simulink model "testemplanner_cs_old"  (R2020b)
settings: Solver=FixedStepAuto  StartTime=0.0  StopTime=50  FixedStep=1/1000  MaxStep=3  RelTol=1e-3
PreLoadFcn:
  | mbxruntime.callbacks.PreLoadFcn(bdroot);
PostLoadFcn:
  | mbxruntime.callbacks.PostLoadFcn(bdroot);
InitFcn:
  | mbxruntime.callbacks.InitFcn(bdroot);
StartFcn:
  | mbxruntime.callbacks.StartFcn(bdroot);
StopFcn:
  | mbxruntime.callbacks.StopFcn(bdroot);
model workspace (MAT data in the model file):
  mbox_table : object (value not decoded)
  model_closed = 0
  sim_status = 0
values from neighbouring files (symbols this model uses):
  c_factor = 43.75    [emplanner_init.m]
  cf = -175016    [emplanner_init.m]
  cr = -130634    [emplanner_init.m]
  global_path_x = [-8.9703 -7.97092389706 -6.97280725051 -5.97596683104 -4.98040839797 -3.98613358222 -2.99314248891 -2.0014346597 -1.01100942869 -0.0218660539602 0.965996233729 1.95257821297 ... (3001 elements, 3001x1)]    [global_path.mat]
  global_path_y = [9.935 9.935 9.935 9.935 9.935 9.935 9.935 9.935 9.935 9.935 9.935 9.935 ... (3001 elements, 3001x1)]    [global_path.mat]
  KD_PID_distance = 0.0    (= 0)    [emplanner_init.m]
  KD_PID_speed = 0    [emplanner_init.m]
  KI_PID_distance = 0.0    (= 0)    [emplanner_init.m]
  KI_PID_speed = 0    [emplanner_init.m]
  KP_PID_distance = 0.5    [emplanner_init.m]
  KP_PID_speed = 1.8    [emplanner_init.m]
  la = 1.265    [emplanner_init.m]
  lb = 2.947-1.265    (= 1.682)    [emplanner_init.m]
  LQR_K1 = k(:,1)'    [emplanner_init.m]
  LQR_K2 = k(:,2)'    [emplanner_init.m]
  LQR_K3 = k(:,3)'    [emplanner_init.m]
  LQR_K4 = k(:,4)'    [emplanner_init.m]
  m = 2020    [emplanner_init.m]
  rack_displacement = [-39.14 , -37.2 , -35.29 , -33.43 , -31.6 , -29.81 , -28.06 , -26.34 , -24.66 ,      -23.01 , -21.38 , -19.79 , -18.23 , -16.69 , -15.18 , -13.7 , -12.23 , -10.8 , -9.38 , -7.98 ,     -6.61 , -5.25 , -3.91 , -2.59 , -1.29 , 0 , 1.27 , 2.54 , 3.78 , 5.02 , 6.24 , 7.46 , 8.66 ,      9.86 , 11.05 , 12.24 , 13.41 , 14.59 , 15.76 , 16.92 , 18.09 , 19.25 , 20.42 , 21.59 , 22.76 ,      23.93 , 25.11 , 26 ...(+26 chars)    [emplanner_init.m]
  right_wheel_ground = [-70 ,-67.2 , -64.4 , -61.6 , -58.8 , -56 , -53.2 , -50.4 , -47.6 , -44.8 , -42 ,      -39.2 , -36.4 , -33.6 , -30.8 , -28 , -25.2 , -22.4 , -19.6 , -16.8 , -14 , -11.2 , -8.4 , -5.6 ,      -2.8 , 0 , 2.8 , 5.6 , 8.4 , 11.2 , 14 , 16.8 , 19.6 , 22.4 , 25.2 , 28 , 30.8 , 33.6 , 36.4 ,      39.2 , 42 , 44.8 , 47.6 , 50.4 , 53.2 , 56 , 58.8 , 61.6 , 64.4 , 67.2 , 70 ]    [emplanner_init.m]
  vx_break_point = zeros(1,5000)    [emplanner_init.m]
undefined symbols (not defined in the file or in its folder): aubr, DiscIntNeverNeededParam, tablebr, vubr, warningInitialVelocity, x0
libraries: PreScanSimulinkLibrary x33, simulink x19, simulink_extras x10, Solver_SF x1
(part 6 of 12)

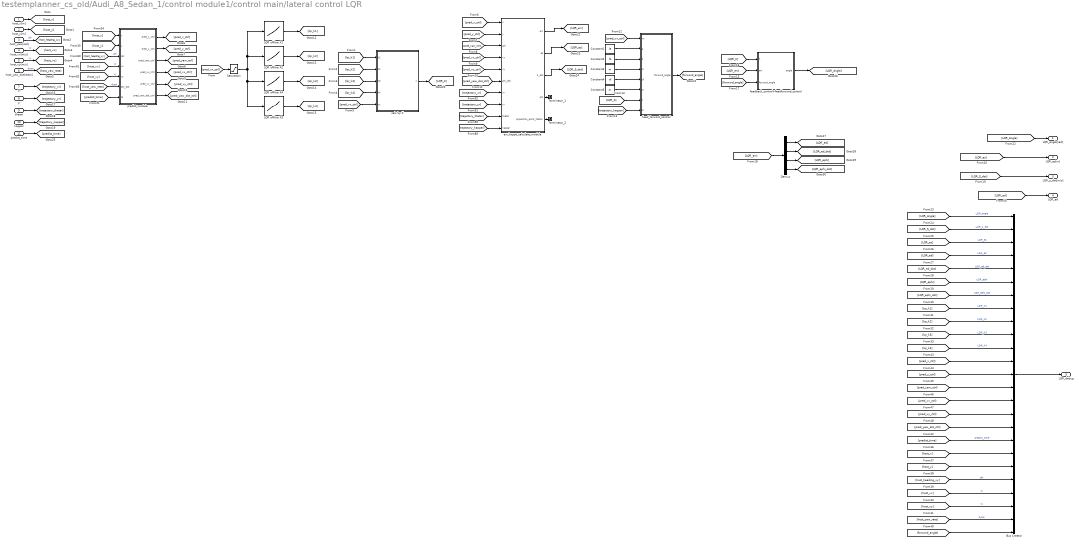
== system testemplanner_cs_old/Audi_A8_Sedan_1/control module1/control main/lateral control LQR ==
  host_x[m] : Inport
  host_y[m] : Inport  Port=2
  host_yaw[rad] : Inport  Port=3
  host_vx[m/s] : Inport  Port=4
  host_vy[m/s] : Inport  Port=5
  host_yaw_dot[rad/s] : Inport  Port=6
  xr : Inport  Port=7
  yr : Inport  Port=8
  thetar : Inport  Port=9
  kappar : Inport  Port=10
  predict_time : Inport  Port=11
  Bus Creator : BusCreator  Inputs=25
  Constant1 : Constant  Value=la
  Constant2 : Constant  Value=lb
  Constant3 : Constant  Value=m
  Constant4 : Constant  Value=cf
  Constant5 : Constant  Value=cr
  Demux : Demux
  LQR offline K1 : Lookup_n-D  NumberOfTableDimensions=1  BreakpointsForDimension1=vx_break_point  Table=LQR_K1  InternalRulePriority=Speed  RndMeth=Simplest  InputSameDT=on
  LQR offline K2 : Lookup_n-D  NumberOfTableDimensions=1  BreakpointsForDimension1=vx_break_point  Table=LQR_K2  InternalRulePriority=Speed  RndMeth=Simplest  InputSameDT=on
  LQR offline K3 : Lookup_n-D  NumberOfTableDimensions=1  BreakpointsForDimension1=vx_break_point  Table=LQR_K3  InternalRulePriority=Speed  RndMeth=Simplest  InputSameDT=on
  LQR offline K4 : Lookup_n-D  NumberOfTableDimensions=1  BreakpointsForDimension1=vx_break_point  Table=LQR_K4  InternalRulePriority=Speed  RndMeth=Simplest  InputSameDT=on
  Saturation : Saturate  UpperLimit=50  LowerLimit=0
  Terminator_1 : Terminator
  Terminator_2 : Terminator
  calc lqr K : MATLAB Function  TreatAsAtomicUnit=on
  err_kappa_calculate_module : MATLAB Function  TreatAsAtomicUnit=on
  feed_forword_control : MATLAB Function  TreatAsAtomicUnit=on
  feedback_control+feedforword_control : MATLAB Function  TreatAsAtomicUnit=on
  predict_module : MATLAB Function  TreatAsAtomicUnit=on
  LQR_angle[rad] : Outport  VectorParamsAs1DForOutWhenUnconnected=off
  LQR_es[m] : Outport  Port=2  VectorParamsAs1DForOutWhenUnconnected=off
  LQR_s_dot[m/s] : Outport  Port=3  VectorParamsAs1DForOutWhenUnconnected=off
  LQR_ed : Outport  Port=4  VectorParamsAs1DForOutWhenUnconnected=off
  LQR_debug : Outport  Port=5  VectorParamsAs1DForOutWhenUnconnected=off
  wires:
  [host_vy] -> predict_module/5(vy)  "vy"
  [host_x] -> predict_module/1(x)
  [host_yaw_rate] -> predict_module/6(phi_dot)  "dyaw"
  [host_vx] -> predict_module/4(vx)  "vx"
  [host_y] -> predict_module/2(y)
  [host_heading_xy] -> predict_module/3(phi)  "phi"
  [predict_time] -> predict_module/7(ts)
  host_x[m]/1 -> [host_x]
  host_y[m]/1 -> [host_y]
  host_yaw[rad]/1 -> [host_heading_xy]  "phi"
  host_vx[m/s]/1 -> [host_vx]  "vx"
  host_vy[m/s]/1 -> [host_vy]  "vy"
  host_yaw_dot[rad/s]/1 -> [host_yaw_rate]  "dyaw"
  predict_module/1(pred_x_ctrl) -> [pred_x_ctrl]
  predict_module/2(pred_y_ctrl) -> [pred_y_ctrl]
  predict_module/3(pred_yaw_ctrl) -> [pred_yaw_ctrl]
  predict_module/4(pred_vx_ctrl) -> [pred_vx_ctrl]
  predict_module/5(pred_vy_ctrl) -> [pred_vy_ctrl]
  predict_module/6(pred_yaw_dot_ctrl) -> [pred_yaw_dot_ctrl]
  [pred_vx_ctrl] -> Saturation/1
  LQR offline K1/1 -> [lqr_k1]
  LQR offline K2/1 -> [lqr_k2]
  LQR offline K4/1 -> [lqr_k3]
  LQR offline K3/1 -> [lqr_k4]
  [pred_vx_ctrl] -> calc lqr K/5(vx)
  [lqr_k4] -> calc lqr K/4(k4)
  [lqr_k3] -> calc lqr K/3(k3)
  [lqr_k2] -> calc lqr K/2(k2)
  [lqr_k1] -> calc lqr K/1(k1)
  [pred_x_ctrl] -> err_kappa_calculate_module/1(x)
  [pred_y_ctrl] -> err_kappa_calculate_module/2(y)
  [pred_yaw_ctrl] -> err_kappa_calculate_module/3("phi ")
  [pred_vx_ctrl] -> err_kappa_calculate_module/4(vx)
  [pred_vy_ctrl] -> err_kappa_calculate_module/5(vy)
  [pred_yaw_dot_ctrl] -> err_kappa_calculate_module/6(phi_dot)
  xr/1 -> [trajectory_xr]
  yr/1 -> [trajectory_yr]
  thetar/1 -> [trajectory_thetar]
  kappar/1 -> [trajectory_kappar]
  [trajectory_xr] -> err_kappa_calculate_module/7(xr)
  [trajectory_yr] -> err_kappa_calculate_module/8(yr)
  [trajectory_kappar] -> err_kappa_calculate_module/10(kappar)
  [trajectory_thetar] -> err_kappa_calculate_module/9(thetar)
  [pred_vx_ctrl] -> feed_forword_control/1(vx)
  Constant1/1 -> feed_forword_control/2(a)
  Constant2/1 -> feed_forword_control/3(b)
  Constant3/1 -> feed_forword_control/4(m)
  Constant4/1 -> feed_forword_control/5(cf)
  Constant5/1 -> feed_forword_control/6(cr)
  calc lqr K/1(k) -> [LQR_K]
  [LQR_K] -> feed_forword_control/7(k)
  [trajectory_kappar] -> feed_forword_control/8(kr)
  feed_forword_control/1(forword_angle) -> [forword_angle]
  err_kappa_calculate_module/1(err) -> [LQR_err]
  [LQR_err] -> feedback_control+feedforword_control/2(err)
  [LQR_K] -> feedback_control+feedforword_control/1(k)
  [forword_angle] -> feedback_control+feedforword_control/3(forword_angle)
  [LQR_err] -> Demux/1
  err_kappa_calculate_module/2(es) -> [LQR_es]
  err_kappa_calculate_module/3(s_dot) -> [LQR_S_dot]
  [LQR_S_dot] -> LQR_s_dot[m/s]/1
  [LQR_es] -> LQR_es[m]/1
  Saturation/1 -> LQR offline K3/1, LQR offline K4/1, LQR offline K2/1, LQR offline K1/1
  predict_time/1 -> [predict_time]
  Bus Creator/1 -> LQR_debug/1
  feedback_control+feedforword_control/1(angle) -> [LQR_Angle]
  [LQR_Angle] -> LQR_angle[rad]/1
  [LQR_Angle] -> Bus Creator/1  "LQR_angle"
  [LQR_S_dot] -> Bus Creator/2  "LQR_s_dot"
  [LQR_es] -> Bus Creator/3  "LQR_es"
  Demux/1 -> [LQR_ed]
  Demux/2 -> [LQR_ed_dot]
  Demux/3 -> [LQR_ephi]
  Demux/4 -> [LQR_ephi_dot]
  [LQR_ed] -> Bus Creator/4  "LQR_ed"
  [LQR_ed_dot] -> Bus Creator/5  "LQR_ed_dot"
  [LQR_ephi] -> Bus Creator/6  "LQR_ephi"
  [LQR_ephi_dot] -> Bus Creator/7  "LQR_ephi_dot"
  [lqr_k1] -> Bus Creator/8  "LQR_K1"
  [lqr_k2] -> Bus Creator/9  "LQR_K2"
  [lqr_k3] -> Bus Creator/10  "LQR_K3"
  [lqr_k4] -> Bus Creator/11  "LQR_K4"
  [pred_x_ctrl] -> Bus Creator/12
  [pred_y_ctrl] -> Bus Creator/13
  [pred_yaw_ctrl] -> Bus Creator/14
  [pred_vx_ctrl] -> Bus Creator/15
  [pred_vy_ctrl] -> Bus Creator/16
  [pred_yaw_dot_ctrl] -> Bus Creator/17
  [predict_time] -> Bus Creator/18  "predict_time"
  [host_x] -> Bus Creator/19
  [host_y] -> Bus Creator/20
  [host_heading_xy] -> Bus Creator/21  "phi"
  [host_vx] -> Bus Creator/22  "vx"
  [host_vy] -> Bus Creator/23  "vy"
  [host_yaw_rate] -> Bus Creator/24  "dyaw"
  [forword_angle] -> Bus Creator/25
  [LQR_ed] -> LQR_ed/1
  err_kappa_calculate_module/4(phi) -> Terminator_1/1
  err_kappa_calculate_module/5(projection_point_thetar) -> Terminator_2/1

== system testemplanner_cs_old/Audi_A8_Sedan_1/control module1/control main/longitudinal control double PID ==
  s_err[m] : Inport
  speed_desire[m/s] : Inport  Port=2
  accelerate desire[m/s^2] : Inport  Port=3
  host_speed[m/s] : Inport  Port=4
  host_s_dot[m/s] : Inport  Port=5
  KP_PID_distance : Inport  Port=6
  KI_PID_distance : Inport  Port=7
  KD_PID_distance : Inport  Port=8
  KP_PID_speed : Inport  Port=9
  KI_PID_speed : Inport  Port=10
  KD_PID_speed : Inport  Port=11
  2-D Lookup Table : Lookup_n-D  BreakpointsForDimension1=vubr  BreakpointsForDimension2=aubr  Table=tablebr  InternalRulePriority=Speed  RndMeth=Simplest  InputSameDT=on
      settings: InputPortMap=u0,u1
  Add : Sum  Inputs=++-
  Add1 : Sum
  Bus Creator : BusCreator  Inputs=9
  Discrete Filter : DiscreteFilter
  MATLAB Function1 : MATLAB Function  TreatAsAtomicUnit=on
  Saturation : Saturate  UpperLimit=45  LowerLimit=-45
  Saturation1 : Saturate  UpperLimit=5  LowerLimit=-8
  discrete pid : Subsystem
  discrete pid1 : Subsystem
  throttle : Outport
  brake : Outport  Port=2
  longitudinal_debug : Outport  Port=3
  wires:
  2-D Lookup Table/1 -> MATLAB Function1/1(u)
  s_err[m]/1 -> [s_err]
  speed_desire[m/s]/1 -> [speed_desire]
  accelerate desire[m/s^2]/1 -> [accelerate_desire]
  KP_PID_distance/1 -> [KP_PID_distance]
  KI_PID_distance/1 -> [KI_PID_distance]
  KD_PID_distance/1 -> [KD_PID_distance]
  KP_PID_speed/1 -> [KP_PID_speed]
  KI_PID_speed/1 -> [KI_PID_speed]
  KD_PID_speed/1 -> [KD_PID_speed]
  [s_err] -> Discrete Filter/1
  host_speed[m/s]/1 -> [host_speed]
  [speed_desire] -> Add/2
  Add/1 -> Saturation/1
  Saturation/1 -> discrete pid1/1(err)
  discrete pid1/1(pid_out) -> Add1/1
  [accelerate_desire] -> Add1/2
  Add1/1 -> Saturation1/1
  Saturation1/1 -> 2-D Lookup Table/2
  host_s_dot[m/s]/1 -> [host_s_dot]
  [host_s_dot] -> Add/3
  [host_speed] -> 2-D Lookup Table/1
  MATLAB Function1/1(throttle) -> throttle/1
  MATLAB Function1/2(brake) -> brake/1
  [KP_PID_distance] -> Bus Creator/1  "KP_PID_distance"
  [KI_PID_distance] -> Bus Creator/2  "KI_PID_distance"
  [KD_PID_distance] -> Bus Creator/3  "KD_PID_distance"
  [KP_PID_speed] -> Bus Creator/4  "KP_PID_speed"
  [KI_PID_speed] -> Bus Creator/5  "KI_PID_speed"
  [KD_PID_speed] -> Bus Creator/6  "KD_PID_speed"
  [host_speed] -> Bus Creator/7  "host_speed"
  [s_err] -> Bus Creator/8  "s_err"
  [host_s_dot] -> Bus Creator/9  "host_s_dot"
  Bus Creator/1 -> longitudinal_debug/1
  Discrete Filter/1 -> discrete pid/1(err)
  [KP_PID_distance] -> discrete pid/2(kp)
  [KI_PID_distance] -> discrete pid/3(ki)
  [KD_PID_distance] -> discrete pid/4(kd)
  [KP_PID_speed] -> discrete pid1/2(kp)
  [KI_PID_speed] -> discrete pid1/3(ki)
  [KD_PID_speed] -> discrete pid1/4(kd)
  discrete pid/1(pid_out) -> Add/1

== system testemplanner_cs_old/Audi_A8_Sedan_1/control module1/control main/understeer compensate ==
  LQR_angle : Inport
  lateral err : Inport  Port=2
  Add : Sum  Inputs=+-
  Gain : Gain  Gain=0.01
  Manual Switch : ManualSwitch
  LQR_final_angle : Outport
  wires:
  lateral err/1 -> Gain/1
  Add/1 -> Manual Switch/2
  Manual Switch/1 -> LQR_final_angle/1
  LQR_angle/1 -> Add/1, Manual Switch/1
  Gain/1 -> Add/2

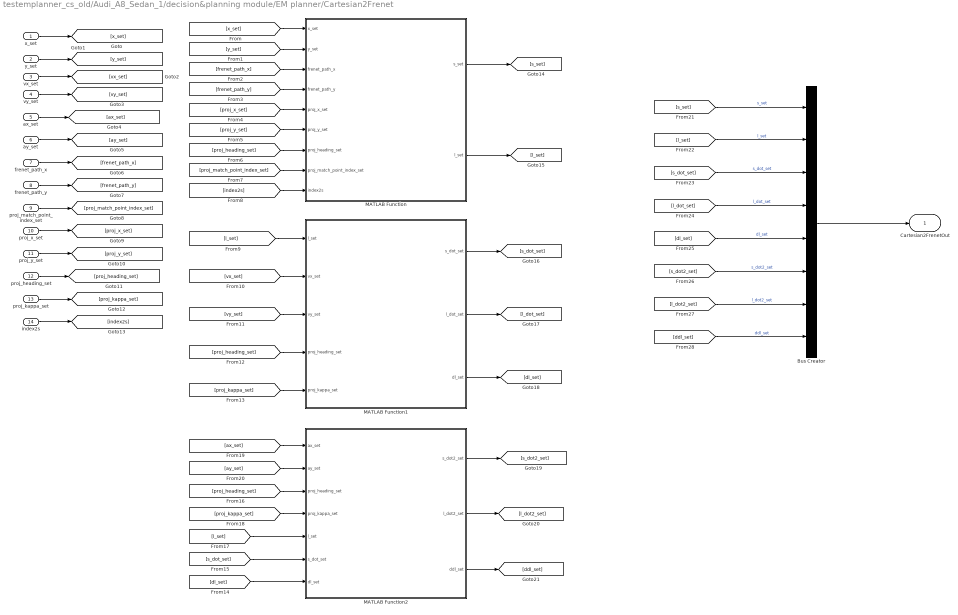
== system testemplanner_cs_old/Audi_A8_Sedan_1/decision&planning module/EM planner/Cartesian2Frenet ==
  x_set : Inport
  y_set : Inport  Port=2
  vx_set : Inport  Port=3
  vy_set : Inport  Port=4
  ax_set : Inport  Port=5
  ay_set : Inport  Port=6
  frenet_path_x : Inport  Port=7
  frenet_path_y : Inport  Port=8
  proj_match_point_index_set : Inport  Port=9
  proj_x_set : Inport  Port=10
  proj_y_set : Inport  Port=11
  proj_heading_set : Inport  Port=12
  proj_kappa_set : Inport  Port=13
  index2s : Inport  Port=14
  Bus Creator : BusCreator  Inputs=8
  MATLAB Function : MATLAB Function  TreatAsAtomicUnit=on
  MATLAB Function1 : MATLAB Function  TreatAsAtomicUnit=on
  MATLAB Function2 : MATLAB Function  TreatAsAtomicUnit=on
  Cartesian2FrenetOut : Outport
  wires:
  x_set/1 -> [x_set]
  y_set/1 -> [y_set]
  vx_set/1 -> [vx_set]
  vy_set/1 -> [vy_set]
  ax_set/1 -> [ax_set]
  ay_set/1 -> [ay_set]
  frenet_path_x/1 -> [frenet_path_x]
  frenet_path_y/1 -> [frenet_path_y]
  proj_match_point_index_set/1 -> [proj_match_point_index_set]
  proj_x_set/1 -> [proj_x_set]
  proj_y_set/1 -> [proj_y_set]
  proj_heading_set/1 -> [proj_heading_set]
  proj_kappa_set/1 -> [proj_kappa_set]
  index2s/1 -> [index2s]
  [index2s] -> MATLAB Function/9(index2s)
  [proj_match_point_index_set] -> MATLAB Function/8(proj_match_point_index_set)
  [proj_heading_set] -> MATLAB Function/7(proj_heading_set)
  [proj_y_set] -> MATLAB Function/6(proj_y_set)
  [proj_x_set] -> MATLAB Function/5(proj_x_set)
  [frenet_path_y] -> MATLAB Function/4(frenet_path_y)
  [frenet_path_x] -> MATLAB Function/3(frenet_path_x)
  [y_set] -> MATLAB Function/2(y_set)
  [x_set] -> MATLAB Function/1(x_set)
  MATLAB Function/1(s_set) -> [s_set]
  MATLAB Function/2(l_set) -> [l_set]
  [l_set] -> MATLAB Function1/1(l_set)
  [vx_set] -> MATLAB Function1/2(vx_set)
  [vy_set] -> MATLAB Function1/3(vy_set)
  [proj_heading_set] -> MATLAB Function1/4(proj_heading_set)
  [proj_kappa_set] -> MATLAB Function1/5(proj_kappa_set)
  MATLAB Function1/1(s_dot_set) -> [s_dot_set]
  MATLAB Function1/3(dl_set) -> [dl_set]
  MATLAB Function1/2(l_dot_set) -> [l_dot_set]
  [dl_set] -> MATLAB Function2/7(dl_set)
  [s_dot_set] -> MATLAB Function2/6(s_dot_set)
  [l_set] -> MATLAB Function2/5(l_set)
  [proj_kappa_set] -> MATLAB Function2/4(proj_kappa_set)
  [proj_heading_set] -> MATLAB Function2/3(proj_heading_set)
  [ax_set] -> MATLAB Function2/1(ax_set)
  [ay_set] -> MATLAB Function2/2(ay_set)
  MATLAB Function2/1(s_dot2_set) -> [s_dot2_set]
  Bus Creator/1 -> Cartesian2FrenetOut/1
  [s_set] -> Bus Creator/1  "s_set"
  [l_set] -> Bus Creator/2  "l_set"
  [s_dot_set] -> Bus Creator/3  "s_dot_set"
  [l_dot_set] -> Bus Creator/4  "l_dot_set"
  [dl_set] -> Bus Creator/5  "dl_set"
  [s_dot2_set] -> Bus Creator/6  "s_dot2_set"
  [l_dot2_set] -> Bus Creator/7  "l_dot2_set"
  [ddl_set] -> Bus Creator/8  "ddl_set"
  MATLAB Function2/2(l_dot2_set) -> [l_dot2_set]
  MATLAB Function2/3(ddl_set) -> [ddl_set]

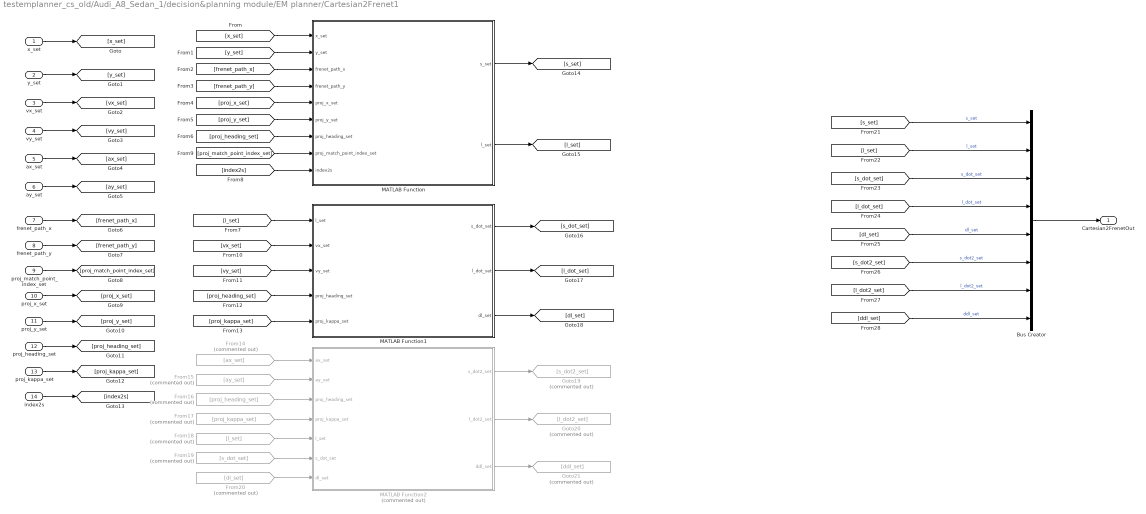
== system testemplanner_cs_old/Audi_A8_Sedan_1/decision&planning module/EM planner/Cartesian2Frenet1 ==
  x_set : Inport
  y_set : Inport  Port=2
  vx_set : Inport  Port=3
  vy_set : Inport  Port=4
  ax_set : Inport  Port=5
  ay_set : Inport  Port=6
  frenet_path_x : Inport  Port=7
  frenet_path_y : Inport  Port=8
  proj_match_point_index_set : Inport  Port=9
  proj_x_set : Inport  Port=10
  proj_y_set : Inport  Port=11
  proj_heading_set : Inport  Port=12
  proj_kappa_set : Inport  Port=13
  index2s : Inport  Port=14
  Bus Creator : BusCreator  Inputs=8
  From14 : From  Commented=on  GotoTag=ax_set
  From15 : From  Commented=on  GotoTag=ay_set
  From16 : From  Commented=on  GotoTag=proj_heading_set
  From17 : From  Commented=on  GotoTag=proj_kappa_set
  From18 : From  Commented=on  GotoTag=l_set
  From19 : From  Commented=on  GotoTag=s_dot_set
  From20 : From  Commented=on  GotoTag=dl_set
  Goto19 : Goto  Commented=on  GotoTag=s_dot2_set
  Goto20 : Goto  Commented=on  GotoTag=l_dot2_set
  Goto21 : Goto  Commented=on  GotoTag=ddl_set
  MATLAB Function : MATLAB Function  TreatAsAtomicUnit=on
  MATLAB Function1 : MATLAB Function  TreatAsAtomicUnit=on
  MATLAB Function2 : MATLAB Function  Commented=on  TreatAsAtomicUnit=on
  Cartesian2FrenetOut : Outport
  wires:
  Bus Creator/1 -> Cartesian2FrenetOut/1
  [ddl_set] -> Bus Creator/8  "ddl_set"
  [l_dot2_set] -> Bus Creator/7  "l_dot2_set"
  [s_dot2_set] -> Bus Creator/6  "s_dot2_set"
  [dl_set] -> Bus Creator/5  "dl_set"
  [l_dot_set] -> Bus Creator/4  "l_dot_set"
  [s_dot_set] -> Bus Creator/3  "s_dot_set"
  [l_set] -> Bus Creator/2  "l_set"
  [s_set] -> Bus Creator/1  "s_set"
  MATLAB Function2/3(ddl_set) -> Goto21/1
  MATLAB Function2/2(l_dot2_set) -> Goto20/1
  MATLAB Function2/1(s_dot2_set) -> Goto19/1
  From20/1 -> MATLAB Function2/7(dl_set)
  From19/1 -> MATLAB Function2/6(s_dot_set)
  MATLAB Function1/3(dl_set) -> [dl_set]
  MATLAB Function1/2(l_dot_set) -> [l_dot_set]
  MATLAB Function1/1(s_dot_set) -> [s_dot_set]
  From18/1 -> MATLAB Function2/5(l_set)
  From17/1 -> MATLAB Function2/4(proj_kappa_set)
  From16/1 -> MATLAB Function2/3(proj_heading_set)
  From15/1 -> MATLAB Function2/2(ay_set)
  From14/1 -> MATLAB Function2/1(ax_set)
  [proj_kappa_set] -> MATLAB Function1/5(proj_kappa_set)
  [proj_heading_set] -> MATLAB Function1/4(proj_heading_set)
  [vy_set] -> MATLAB Function1/3(vy_set)
  [vx_set] -> MATLAB Function1/2(vx_set)
  [l_set] -> MATLAB Function1/1(l_set)
  MATLAB Function/2(l_set) -> [l_set]
  MATLAB Function/1(s_set) -> [s_set]
  [index2s] -> MATLAB Function/9(index2s)
  [proj_heading_set] -> MATLAB Function/7(proj_heading_set)
  [proj_y_set] -> MATLAB Function/6(proj_y_set)
  [proj_match_point_index_set] -> MATLAB Function/8(proj_match_point_index_set)
  [proj_x_set] -> MATLAB Function/5(proj_x_set)
  [frenet_path_y] -> MATLAB Function/4(frenet_path_y)
  [frenet_path_x] -> MATLAB Function/3(frenet_path_x)
  [y_set] -> MATLAB Function/2(y_set)
  [x_set] -> MATLAB Function/1(x_set)
  index2s/1 -> [index2s]
  proj_kappa_set/1 -> [proj_kappa_set]
  proj_heading_set/1 -> [proj_heading_set]
  proj_y_set/1 -> [proj_y_set]
  proj_x_set/1 -> [proj_x_set]
  proj_match_point_index_set/1 -> [proj_match_point_index_set]
  frenet_path_y/1 -> [frenet_path_y]
  frenet_path_x/1 -> [frenet_path_x]
  ay_set/1 -> [ay_set]
  ax_set/1 -> [ax_set]
  vy_set/1 -> [vy_set]
  vx_set/1 -> [vx_set]
  y_set/1 -> [y_set]
  x_set/1 -> [x_set]

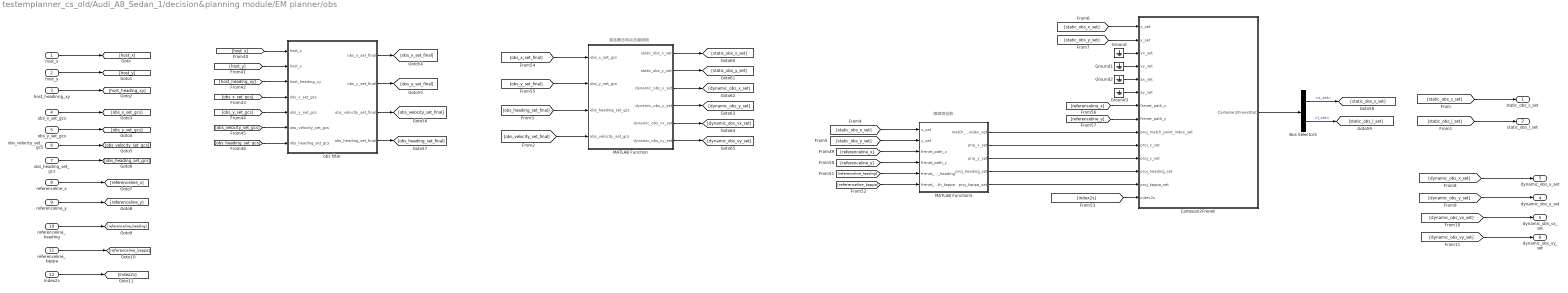
== system testemplanner_cs_old/Audi_A8_Sedan_1/decision&planning module/EM planner/obs ==
  note: 筛选静态和动态障碍物
  note: 障碍物投影
  host_x : Inport
  host_y : Inport  Port=2
  host_headinng_xy : Inport  Port=3
  obs_x_set_gcs : Inport  Port=4
  obs_y_set_gcs : Inport  Port=5
  obs_velocity_set_gcs : Inport  Port=6
  obs_heading_set_gcs : Inport  Port=7
  referenceline_x : Inport  Port=8
  referenceline_y : Inport  Port=9
  referenceline_heading : Inport  Port=10
  referenceline_kappa : Inport  Port=11
  index2s : Inport  Port=12
  Bus Selector5 : BusSelector  OutputSignals=s_set,l_set
  Cartesian2Frenet : Subsystem
  Ground{,1..3} (4 alike) : Ground
  MATLAB Function : MATLAB Function  TreatAsAtomicUnit=on
  MATLAB Function5 : MATLAB Function  TreatAsAtomicUnit=on
  obs filter : MATLAB Function  TreatAsAtomicUnit=on
  static_obs_s_set : Outport
  static_obs_l_set : Outport  Port=2
  dynamic_obs_x_set : Outport  Port=3
  dynamic_obs_y_set : Outport  Port=4
  dynamic_obs_vx_set : Outport  Port=5
  dynamic_obs_vy_set : Outport  Port=6
  wires:
  [obs_heading_set_final] -> MATLAB Function/3(obs_heading_set_gcs)
  [host_x] -> obs filter/1(host_x)
  obs filter/3(obs_velocity_set_final) -> [obs_velocity_set_final]
  Ground3/1 -> Cartesian2Frenet/6(ay_set)
  [referenceline_y] -> MATLAB Function5/4(frenet_path_y)
  [obs_x_set_gcs] -> obs filter/4(obs_x_set_gcs)
  [static_obs_x_set] -> Cartesian2Frenet/1(x_set)
  [referenceline_y] -> Cartesian2Frenet/8(frenet_path_y)
  obs filter/2(obs_y_set_final) -> [obs_y_set_final]
  obs filter/1(obs_x_set_final) -> [obs_x_set_final]
  Ground/1 -> Cartesian2Frenet/3(vx_set)
  MATLAB Function/1(static_obs_x_set) -> [static_obs_x_set]
  Ground1/1 -> Cartesian2Frenet/4(vy_set)
  MATLAB Function/3(dynamic_obs_x_set) -> [dynamic_obs_x_set]
  MATLAB Function5/5(proj_kappa_set) -> Cartesian2Frenet/13(proj_kappa_set)
  [obs_heading_set_gcs] -> obs filter/7(obs_heading_set_gcs)
  Ground2/1 -> Cartesian2Frenet/5(ax_set)
  [referenceline_kappa] -> MATLAB Function5/6(frenet_path_kappa)
  [host_y] -> obs filter/2(host_y)
  Cartesian2Frenet/1(Cartesian2FrenetOut) -> Bus Selector5/1
  [referenceline_x] -> Cartesian2Frenet/7(frenet_path_x)
  MATLAB Function5/4(proj_heading_set) -> Cartesian2Frenet/12(proj_heading_set)
  [host_heading_xy] -> obs filter/3(host_heading_xy)
  Bus Selector5/1 -> [static_obs_s_set]  "<s_set>"
  [obs_y_set_gcs] -> obs filter/5(obs_y_set_gcs)
  [static_obs_y_set] -> Cartesian2Frenet/2(y_set)
  [referenceline_heading] -> MATLAB Function5/5(frenet_path_heading)
  obs filter/4(obs_heading_set_final) -> [obs_heading_set_final]
  [obs_x_set_final] -> MATLAB Function/1(obs_x_set_gcs)
  [obs_velocity_set_gcs] -> obs filter/6(obs_velocity_set_gcs)
  MATLAB Function5/3(proj_y_set) -> Cartesian2Frenet/11(proj_y_set)
  [static_obs_y_set] -> MATLAB Function5/2(y_set)
  MATLAB Function5/2(proj_x_set) -> Cartesian2Frenet/10(proj_x_set)
  MATLAB Function/5(dynamic_obs_vx_set) -> [dynamic_obs_vx_set]
  MATLAB Function5/1(match_point_index_set) -> Cartesian2Frenet/9(proj_match_point_index_set)
  MATLAB Function/2(static_obs_y_set) -> [static_obs_y_set]
  Bus Selector5/2 -> [static_obs_l_set]  "<l_set>"
  MATLAB Function/6(dynamic_obs_vy_set) -> [dynamic_obs_vy_set]
  [referenceline_x] -> MATLAB Function5/3(frenet_path_x)
  [index2s] -> Cartesian2Frenet/14(index2s)
  [static_obs_x_set] -> MATLAB Function5/1(x_set)
  MATLAB Function/4(dynamic_obs_y_set) -> [dynamic_obs_y_set]
  [obs_velocity_set_final] -> MATLAB Function/4(obs_velocity_set_gcs)
  [obs_y_set_final] -> MATLAB Function/2(obs_y_set_gcs)
  host_x/1 -> [host_x]
  host_y/1 -> [host_y]
  host_headinng_xy/1 -> [host_heading_xy]
  obs_x_set_gcs/1 -> [obs_x_set_gcs]
  obs_y_set_gcs/1 -> [obs_y_set_gcs]
  obs_velocity_set_gcs/1 -> [obs_velocity_set_gcs]
  obs_heading_set_gcs/1 -> [obs_heading_set_gcs]
  referenceline_x/1 -> [referenceline_x]
  referenceline_heading/1 -> [referenceline_heading]
  referenceline_kappa/1 -> [referenceline_kappa]
  referenceline_y/1 -> [referenceline_y]
  [static_obs_s_set] -> static_obs_s_set/1
  [static_obs_l_set] -> static_obs_l_set/1
  index2s/1 -> [index2s]
  [dynamic_obs_y_set] -> dynamic_obs_y_set/1
  [dynamic_obs_vx_set] -> dynamic_obs_vx_set/1
  [dynamic_obs_x_set] -> dynamic_obs_x_set/1
  [dynamic_obs_vy_set] -> dynamic_obs_vy_set/1

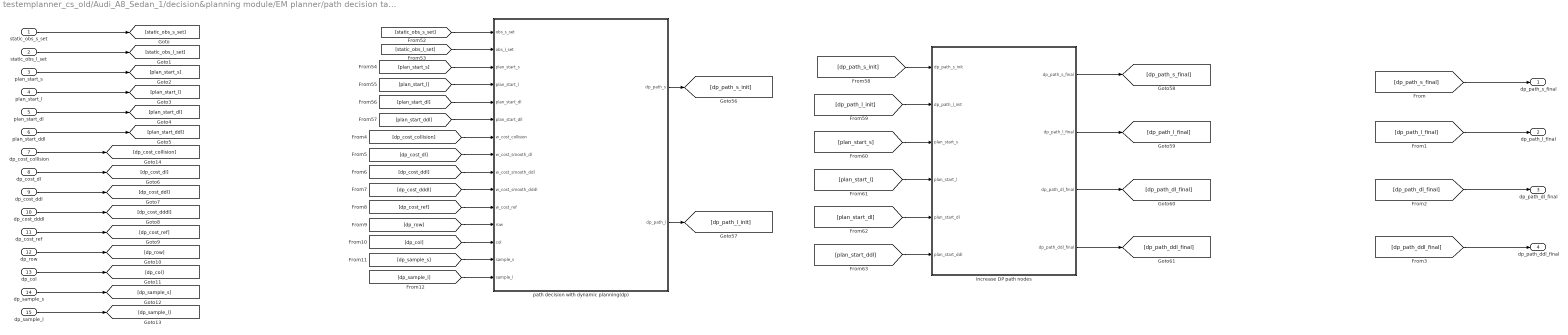
== system testemplanner_cs_old/Audi_A8_Sedan_1/decision&planning module/EM planner/path decision task ==
  static_obs_s_set : Inport
  static_obs_l_set : Inport  Port=2
  plan_start_s : Inport  Port=3
  plan_start_l : Inport  Port=4
  plan_start_dl : Inport  Port=5
  plan_start_ddl : Inport  Port=6
  dp_cost_collision : Inport  Port=7
  dp_cost_dl : Inport  Port=8
  dp_cost_ddl : Inport  Port=9
  dp_cost_dddl : Inport  Port=10
  dp_cost_ref : Inport  Port=11
  dp_row : Inport  Port=12
  dp_col : Inport  Port=13
  dp_sample_s : Inport  Port=14
  dp_sample_l : Inport  Port=15
  increase DP path nodes : MATLAB Function  TreatAsAtomicUnit=on
  path decision with dynamic planning(dp) : MATLAB Function  TreatAsAtomicUnit=on
  dp_path_s_final : Outport
  dp_path_l_final : Outport  Port=2
  dp_path_dl_final : Outport  Port=3
  dp_path_ddl_final : Outport  Port=4
  wires:
  [plan_start_s] -> path decision with dynamic planning(dp)/3(plan_start_s)
  path decision with dynamic planning(dp)/1(dp_path_s) -> [dp_path_s_init]
  increase DP path nodes/2(dp_path_l_final) -> [dp_path_l_final]
  [static_obs_l_set] -> path decision with dynamic planning(dp)/2(obs_l_set)
  [plan_start_ddl] -> path decision with dynamic planning(dp)/6(plan_start_dll)
  [plan_start_l] -> path decision with dynamic planning(dp)/4(plan_start_l)
  [static_obs_s_set] -> path decision with dynamic planning(dp)/1(obs_s_set)
  [plan_start_dl] -> increase DP path nodes/5(plan_start_dl)
  increase DP path nodes/4(dp_path_ddl_final) -> [dp_path_ddl_final]
  increase DP path nodes/1(dp_path_s_final) -> [dp_path_s_final]
  increase DP path nodes/3(dp_path_dl_final) -> [dp_path_dl_final]
  path decision with dynamic planning(dp)/2(dp_path_l) -> [dp_path_l_init]
  [plan_start_l] -> increase DP path nodes/4(plan_start_l)
  [plan_start_ddl] -> increase DP path nodes/6(plan_start_ddl)
  [plan_start_dl] -> path decision with dynamic planning(dp)/5(plan_start_dl)
  [plan_start_s] -> increase DP path nodes/3(plan_start_s)
  [dp_path_l_init] -> increase DP path nodes/2(dp_path_l_init)
  [dp_path_s_init] -> increase DP path nodes/1(dp_path_s_init)
  static_obs_s_set/1 -> [static_obs_s_set]
  static_obs_l_set/1 -> [static_obs_l_set]
  plan_start_s/1 -> [plan_start_s]
  plan_start_l/1 -> [plan_start_l]
  plan_start_dl/1 -> [plan_start_dl]
  plan_start_ddl/1 -> [plan_start_ddl]
  [dp_path_s_final] -> dp_path_s_final/1
  [dp_path_l_final] -> dp_path_l_final/1
  [dp_path_dl_final] -> dp_path_dl_final/1
  [dp_path_ddl_final] -> dp_path_ddl_final/1
  [dp_cost_collision] -> path decision with dynamic planning(dp)/7(w_cost_collision)
  [dp_cost_dl] -> path decision with dynamic planning(dp)/8(w_cost_smooth_dl)
  [dp_cost_ddl] -> path decision with dynamic planning(dp)/9(w_cost_smooth_ddl)
  [dp_cost_dddl] -> path decision with dynamic planning(dp)/10(w_cost_smooth_dddl)
  [dp_cost_ref] -> path decision with dynamic planning(dp)/11(w_cost_ref)
  [dp_row] -> path decision with dynamic planning(dp)/12(row)
  [dp_col] -> path decision with dynamic planning(dp)/13(col)
  [dp_sample_s] -> path decision with dynamic planning(dp)/14(sample_s)
  [dp_sample_l] -> path decision with dynamic planning(dp)/15(sample_l)
  dp_cost_dl/1 -> [dp_cost_dl]
  dp_cost_ddl/1 -> [dp_cost_ddl]
  dp_cost_dddl/1 -> [dp_cost_dddl]
  dp_cost_ref/1 -> [dp_cost_ref]
  dp_row/1 -> [dp_row]
  dp_col/1 -> [dp_col]
  dp_sample_l/1 -> [dp_sample_l]
  dp_sample_s/1 -> [dp_sample_s]
  dp_cost_collision/1 -> [dp_cost_collision]

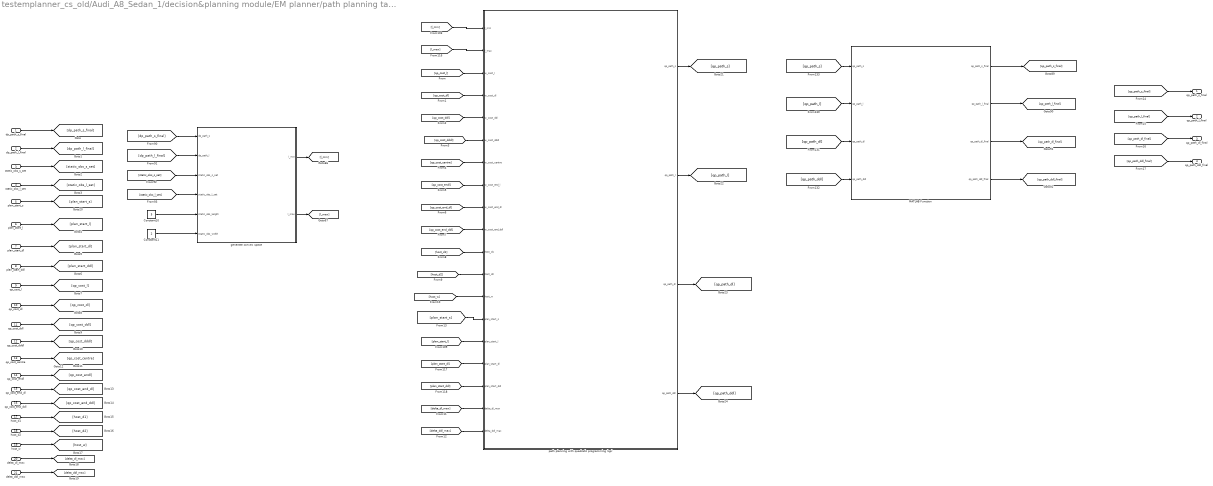
== system testemplanner_cs_old/Audi_A8_Sedan_1/decision&planning module/EM planner/path planning task ==
  dp_path_s_final : Inport
  dp_path_l_final : Inport  Port=2
  static_obs_s_set : Inport  Port=3
  static_obs_l_set : Inport  Port=4
  plan_start_s : Inport  Port=5
  plan_start_l : Inport  Port=6
  plan_start_dl : Inport  Port=7
  plan_start_ddl : Inport  Port=8
  qp_cost_l : Inport  Port=9
  qp_cost_dl : Inport  Port=10
  qp_cost_ddl : Inport  Port=11
  qp_cost_dddl : Inport  Port=12
  qp_cost_centre : Inport  Port=13
  qp_cost_endl : Inport  Port=14
  qp_cost_end_dl : Inport  Port=15
  qp_cost_end_ddl : Inport  Port=16
  host_d1 : Inport  Port=17
  host_d2 : Inport  Port=18
  host_w : Inport  Port=19
  delta_dl_max : Inport  Port=20
  delta_ddl_max : Inport  Port=21
  Constant10 : Constant  Value=5
  Constant11 : Constant  Value=2
  MATLAB Function : MATLAB Function  TreatAsAtomicUnit=on
  generate convex space : MATLAB Function  TreatAsAtomicUnit=on
  path planning with quadratic programming (qp) : MATLAB Function  TreatAsAtomicUnit=on
  qp_path_s_final : Outport
  qp_path_l_final : Outport  Port=2
  qp_path_dl_final : Outport  Port=3
  qp_path_ddl_final : Outport  Port=4
  wires:
  generate convex space/2(l_max) -> [l_max]
  Constant11/1 -> generate convex space/6(static_obs_width)
  Constant10/1 -> generate convex space/5(static_obs_length)
  [static_obs_l_set] -> generate convex space/4(static_obs_l_set)
  [dp_path_s_final] -> generate convex space/1(dp_path_s)
  [plan_start_l] -> path planning with quadratic programming (qp)/15(plan_start_l)
  generate convex space/1(l_min) -> [l_min]
  [static_obs_s_set] -> generate convex space/3(static_obs_s_set)
  [dp_path_l_final] -> generate convex space/2(dp_path_l)
  [plan_start_dl] -> path planning with quadratic programming (qp)/16(plan_start_dl)
  [l_max] -> path planning with quadratic programming (qp)/2(l_max)
  [l_min] -> path planning with quadratic programming (qp)/1(l_min)
  [plan_start_ddl] -> path planning with quadratic programming (qp)/17(plan_start_ddl)
  dp_path_s_final/1 -> [dp_path_s_final]
  dp_path_l_final/1 -> [dp_path_l_final]
  static_obs_s_set/1 -> [static_obs_s_set]
  static_obs_l_set/1 -> [static_obs_l_set]
  plan_start_l/1 -> [plan_start_l]
  plan_start_dl/1 -> [plan_start_dl]
  plan_start_ddl/1 -> [plan_start_ddl]
  [qp_cost_l] -> path planning with quadratic programming (qp)/3(w_cost_l)
  [qp_cost_dl] -> path planning with quadratic programming (qp)/4(w_cost_dl)
  [qp_cost_ddl] -> path planning with quadratic programming (qp)/5(w_cost_ddl)
  [qp_cost_dddl] -> path planning with quadratic programming (qp)/6(w_cost_dddl)
  [qp_cost_centre] -> path planning with quadratic programming (qp)/7(w_cost_centre)
  [qp_cost_endl] -> path planning with quadratic programming (qp)/8(w_cost_end_l)
  [qp_cost_end_dl] -> path planning with quadratic programming (qp)/9(w_cost_end_dl)
  [qp_cost_end_ddl] -> path planning with quadratic programming (qp)/10(w_cost_end_ddl)
  [host_d1] -> path planning with quadratic programming (qp)/11(host_d1)
  [host_d2] -> path planning with quadratic programming (qp)/12(host_d2)
  [host_w] -> path planning with quadratic programming (qp)/13(host_w)
  qp_cost_l/1 -> [qp_cost_l]
  qp_cost_dl/1 -> [qp_cost_dl]
  qp_cost_ddl/1 -> [qp_cost_ddl]
  qp_cost_dddl/1 -> [qp_cost_dddl]
  qp_cost_centre/1 -> [qp_cost_centre]
  qp_cost_endl/1 -> [qp_cost_endl]
  qp_cost_end_dl/1 -> [qp_cost_end_dl]
  qp_cost_end_ddl/1 -> [qp_cost_end_ddl]
  host_d1/1 -> [host_d1]
  host_d2/1 -> [host_d2]
  host_w/1 -> [host_w]
  [delta_dl_max] -> path planning with quadratic programming (qp)/18(delta_dl_max)
  [delta_ddl_max] -> path planning with quadratic programming (qp)/19(delta_ddl_max)
  delta_dl_max/1 -> [delta_dl_max]
  delta_ddl_max/1 -> [delta_ddl_max]
  plan_start_s/1 -> [plan_start_s]
  [plan_start_s] -> path planning with quadratic programming (qp)/14(plan_start_s)
  MATLAB Function/1(qp_path_s_final) -> [qp_path_s_final]
  MATLAB Function/3(qp_path_dl_final) -> [qp_path_dl_final]
  [qp_path_s] -> MATLAB Function/1(qp_path_s)
  [qp_path_ddl] -> MATLAB Function/4(qp_path_ddl)
  MATLAB Function/2(qp_path_l_final) -> [qp_path_l_final]
  [qp_path_dl] -> MATLAB Function/3(qp_path_dl)
  MATLAB Function/4(qp_path_ddl_final) -> [qp_path_ddl_final]
  [qp_path_l] -> MATLAB Function/2(qp_path_l)
  [qp_path_s_final] -> qp_path_s_final/1
  [qp_path_l_final] -> qp_path_l_final/1
  [qp_path_dl_final] -> qp_path_dl_final/1
  [qp_path_ddl_final] -> qp_path_ddl_final/1
  path planning with quadratic programming (qp)/1(qp_path_s) -> [qp_path_s]
  path planning with quadratic programming (qp)/2(qp_path_l) -> [qp_path_l]
  path planning with quadratic programming (qp)/3(qp_path_dl) -> [qp_path_dl]
  path planning with quadratic programming (qp)/4(qp_path_ddl) -> [qp_path_ddl]

== system testemplanner_cs_old/Audi_A8_Sedan_2/Dynamics_Simple/Chassis/Bicycle_model_[XYZ] ==
  DeltaWheel_[rad] : Inport
  zFront_[m]_dzFront_[ms-1] : Inport  Port=2  PortDimensions=2
  zRear_[m]_dzRear_[ms-1] : Inport  Port=3  PortDimensions=2
  BrakePressure_[bar] : Inport  Port=4
  DriveTorque_[Nm] : Inport  Port=5
  v0_[ms-1] : Inport  Port=6
  |vx|_[ms-1] : Inport  Port=7
  Fy_rear_[N] : Inport  Port=8
  Fy_front_[N] : Inport  Port=9
  Demux : Demux  Outputs=2
  Demux1 : Demux  Outputs=2
  Fyi --> Fy / Mz : Subsystem
  X_Motion : Subsystem
  Y & Yaw_Motion : Subsystem
  "Z, Pitch_Motion & Roll_Motion" : Subsystem
  |vx|_[ms-1]1 : Outport
  vy_[ms-1] : Outport  Port=2
  vz_[ms-1] : Outport  Port=3
  RollAngle_[rad] : Outport  Port=4
  RollRate_[rads-1] : Outport  Port=5
  YawAngle_[rads-1] : Outport  Port=6
  Vx_[ms-1] : Outport  Port=7
  PitchAngle_[rad] : Outport  Port=8
  YawAngle_[rad] : Outport  Port=9
  ax_[ms-2] : Outport  Port=10
  ay_[ms-2] : Outport  Port=11
  wires:
  Fyi --> Fy / Mz/1(Fy_[N]) -> Y & Yaw_Motion/2(Fy_[N])  "Fy_[N]"
  Fyi --> Fy / Mz/2(Mz_[Nm]) -> Y & Yaw_Motion/3(Mz_[Nm])  "Mz_[Nm]"
  Y & Yaw_Motion/1(|vx|_[ms-1]1) -> |vx|_[ms-1]1/1  "|vx|_[ms-1]"
  Y & Yaw_Motion/2(vy_[ms-1]) -> vy_[ms-1]/1  "vy_[ms-1]"
  Y & Yaw_Motion/5(YawAngle_[rad]) -> YawAngle_[rad]/1  "YawAngle_[rad]"
  v0_[ms-1]/1 -> X_Motion/3(v0_[ms-1])  "v0_[ms-1]"
  BrakePressure_[bar]/1 -> X_Motion/2(BrakePressure_[bar])  "BrakePressure_[bar]"
  DriveTorque_[Nm]/1 -> X_Motion/1(DriveTorque_[Nm])  "DriveTorque_[Nm]"
  X_Motion/2(ax_[ms-2]) -> ax_[ms-2]/1, [ax]  "ax_[ms-2]"
  X_Motion/1(vx_[ms-1]) -> Vx_[ms-1]/1, [vx]  "vx_[ms-1]"
  [ax] -> "Z, Pitch_Motion & Roll_Motion"/3(ax)
  Demux/1 -> "Z, Pitch_Motion & Roll_Motion"/5(zFront_[m])
  Demux/2 -> "Z, Pitch_Motion & Roll_Motion"/6(dzFront_[ms-1])
  Demux1/1 -> "Z, Pitch_Motion & Roll_Motion"/7(zRear_[m])
  Demux1/2 -> "Z, Pitch_Motion & Roll_Motion"/8(dzRear_[ms-1])
  zRear_[m]_dzRear_[ms-1]/1 -> Demux1/1
  zFront_[m]_dzFront_[ms-1]/1 -> Demux/1
  "Z, Pitch_Motion & Roll_Motion"/2(vz_[ms-1]) -> vz_[ms-1]/1  "vz_[ms-1]"
  DeltaWheel_[rad]/1 -> Fyi --> Fy / Mz/1(DeltaWheel_[rad])
  Fy_front_[N]/1 -> Fyi --> Fy / Mz/2(Fy_f_[N])
  Fy_rear_[N]/1 -> Fyi --> Fy / Mz/3(Fy_r_[N])
  |vx|_[ms-1]/1 -> Y & Yaw_Motion/1(|vx|_[ms-1])
  Y & Yaw_Motion/3(ay_[ms-2]) -> [ay], ay_[ms-2]/1  "ay_[ms-2]"
  [ay] -> "Z, Pitch_Motion & Roll_Motion"/4(ay)
  "Z, Pitch_Motion & Roll_Motion"/3(RollAngle_[rad]) -> RollAngle_[rad]/1  "RollAngle_[rad]"
  "Z, Pitch_Motion & Roll_Motion"/4(RollRate_[rads-1]) -> RollRate_[rads-1]/1  "RollRate_[rads-1]"
  [dYaw] -> "Z, Pitch_Motion & Roll_Motion"/2(dYaw)
  [vx] -> "Z, Pitch_Motion & Roll_Motion"/1(vx)
  Y & Yaw_Motion/4(dYawAngle_[rads-1]) -> YawAngle_[rads-1]/1, [dYaw]  "dYawAngle_[rads-1]"
  "Z, Pitch_Motion & Roll_Motion"/1(pitchAngle_[rad]) -> PitchAngle_[rad]/1  "PitchAngle_[rad]"

== system testemplanner_cs_old/Audi_A8_Sedan_2/Dynamics_Simple/Chassis/FrontTyre ==
  note: alpha limiter
      | [-1 ... 1]
  note: relax_on
      | ON: 1
      | OFF: 0
  note: MOTORCYCLE ONLY
  note: VEHICLE + MOTORCYCLE
  DeltaWheel_[rad] : Inport
  |vx|_[ms-1] : Inport  Port=2
  vy_[ms-1] : Inport  Port=3
  dYawAngle_[rads-1] : Inport  Port=4
  RollAngle_[rad] : Inport  Port=5
  AlphaFront : Subsystem
  Compare To Zero : simulink/Logic and Bit Operations/Compare To Zero  relop===  OutDataTypeStr=boolean  ZeroCross=off
  Configurable Subsystem : Subsystem  BlockChoice=Integrator  mask{ComputationMode=ComputationMode}
      mask prompts: ComputationMode "Computation mode:"
      mask init:
      | SetComputationMode(gcb,ComputationMode);
      settings: AttributesFormatString=%<BlockChoice>  OpenFcn=BringToFront(gcb);  MemberBlocks=Discrete-Time Integrator,Integrator
      settings: TemplateBlock=|
      | PreScanSimulinkLibrary/Configurable Subsystems/integral with reset and limits
      | for slip angle/Configurable
      | Subsystem
  Configurable Subsystem1 : Subsystem  BlockChoice=Integrator  mask{ComputationMode=ComputationMode}
      mask prompts: ComputationMode "Computation mode:"
      mask init:
      | SetComputationMode(gcb,ComputationMode);
      settings: AttributesFormatString=%<BlockChoice>  OpenFcn=BringToFront(gcb);  MemberBlocks=Discrete-Time Integrator,Integrator
      settings: TemplateBlock=|
      | PreScanSimulinkLibrary/Configurable Subsystems/integral with reset/Configurable
      | Subsystem
  Constant : Constant  Value=p.relax_on
  Constant1 : Constant  Value=p.relax_on
  Constant2 : Constant  Value=p.VehMCSwitch
  Data Type Conversion : DataTypeConversion  OutDataTypeStr=double
  If MC : simulink/Logic and Bit Operations/Compare To Constant  relop===  const=2  OutDataTypeStr=uint8  ZeroCross=off
  K_gamma_front : Gain  Gain=p.Kgfront
  Linl : Fcn  Expr=(u(4) - u(5))/p.sigma_front*u(1)
  Linl1 : Fcn  Expr=(u(4) - u(5))/p.sigma_front*u(1)
  Mux1 : Mux  Inputs=3
  Mux2 : Mux  Inputs={3,1,1}
  Mux3 : Mux  Inputs={3,1,1}
  Prevent_instability_at_low_Vx : Subsystem
  Product : Product  RndMeth=Zero
  Sum : Sum  Inputs=|++  InputSameDT=on  SaturateOnIntegerOverflow=on  OutDataTypeStr=Inherit: Same as first input
  Sum1 : Sum  Inputs=|++
  Switch : Switch  Threshold=0.5  SaturateOnIntegerOverflow=on  InputSameDT=on
  Switch1 : Switch  Threshold=0.5  SaturateOnIntegerOverflow=on  InputSameDT=on
  alg.loop : Memory
  due to sign convention : Gain  Gain=-1  SaturateOnIntegerOverflow=on  OutDataTypeStr=Inherit: Same as input  ParamDataTypeStr=Inherit: Same as input
  front_tyre : Gain  Gain=p.Kfront
  FyFront_[N] : Outport
  wires:
  Prevent_instability_at_low_Vx/1(alpha [rad]) -> Mux2/2, Switch/3
  Sum/1 -> Prevent_instability_at_low_Vx/1(alpha[rad])  "AlphaStatFront_[rad]"
  Switch/1 -> front_tyre/1  "AlphaFront_[rad]"
  Constant/1 -> Switch/2
  Sum1/1 -> FyFront_[N]/1  "FyFront_[N]"
  Mux2/1 -> Linl/1
  Linl/1 -> Configurable Subsystem/1(In1)
  Configurable Subsystem/1(Out1) -> Mux2/3, Switch/1  "AlphaRelaxFront_[rad]"
  AlphaFront/1(Alpha) -> Sum/1
  Mux1/1 -> Prevent_instability_at_low_Vx/2(In), AlphaFront/1(In), Mux2/1, Mux3/1
  |vx|_[ms-1]/1 -> Mux1/1, Compare To Zero/1
  vy_[ms-1]/1 -> Mux1/2
  dYawAngle_[rads-1]/1 -> Mux1/3
  alg.loop/1 -> Switch1/3
  Configurable Subsystem1/1(Out1) -> Mux3/3, Switch1/1  "GammaRelaxFront_[rad]"
  Linl1/1 -> Configurable Subsystem1/1(In1)
  Mux3/1 -> Linl1/1
  Constant1/1 -> Switch1/2
  due to sign convention/1 -> alg.loop/1, Mux3/2  "GammaStatFront_[rad]"
  RollAngle_[rad]/1 -> due to sign convention/1
  front_tyre/1 -> Sum1/1
  Constant2/1 -> If MC/1
  If MC/1 -> Data Type Conversion/1
  K_gamma_front/1 -> Product/1
  Product/1 -> Sum1/2
  Data Type Conversion/1 -> Product/2
  Compare To Zero/1 -> [reset]
  [reset] -> Configurable Subsystem/2(In2)
  [reset] -> Configurable Subsystem1/2(In2)
  DeltaWheel_[rad]/1 -> Sum/2  "DeltaWheel_[rad]"
  Switch1/1 -> K_gamma_front/1  "GammaFront_[rad]"

== system testemplanner_cs_old/Audi_A8_Sedan_2/Dynamics_Simple/Chassis/MuxDynState ==
  note: The position inputs are computed by the
      | integrated velocity.
  note: mode: Dynamics
      | VelVEHICLE
      | wrt VEH
  note: AnglesVEHICLE
      | wrtGLOB
  vx [ms-1] : Inport
  vy [ms-1] : Inport  Port=2
  vz [ms-1] : Inport  Port=3
  R [rad] : Inport  Port=4
  P [rad] : Inport  Port=5
  Y [rad] : Inport  Port=6
  Configurable Subsystem1 : Subsystem  BlockChoice=Integrator  mask{ComputationMode=ComputationMode}
      mask prompts: ComputationMode "Computation mode:"
      mask init:
      | SetComputationMode(gcb,ComputationMode);
      settings: AttributesFormatString=%<BlockChoice>  OpenFcn=BringToFront(gcb);  MemberBlocks=Discrete-Time Integrator,Integrator
      settings: TemplateBlock=|
      | PreScanSimulinkLibrary/Configurable Subsystems/integral/Configurable
      | Subsystem1
  Ground : Ground
  Ground1 : Ground
  Mux : Mux  Inputs=[3 3 3]
  Mux1 : Mux  Inputs=3
  Mux2 : Mux  Inputs=3
  Transformation_BODY2GLOBAL : Subsystem
  mux3 : Mux  Inputs=3
  State : Outport
  wires:
  Ground1/1 -> mux3/2  "pitch"
  Y [rad]/1 -> Mux2/3, mux3/3  "yaw"
  P [rad]/1 -> Mux2/2
  R [rad]/1 -> Mux2/1
  vz [ms-1]/1 -> Mux1/3
  vy [ms-1]/1 -> Mux1/2
  vx [ms-1]/1 -> Mux1/1
  Mux2/1 -> Mux/3
  Transformation_BODY2GLOBAL/1(Vvector_GLOBAL_[m/s]) -> Configurable Subsystem1/1(In1), Mux/2  "VelVEH wrt  GLOB"
  mux3/1 -> Transformation_BODY2GLOBAL/2(angles_BODYwrtGLOB_[rad])
  Ground/1 -> mux3/1  "roll"
  Mux/1 -> State/1
  Mux1/1 -> Transformation_BODY2GLOBAL/1(Vvector_BODY_[m/s])
  Configurable Subsystem1/1(Out1) -> Mux/1  "PosVEH wrt  GLOB"

== system testemplanner_cs_old/Audi_A8_Sedan_2/Dynamics_Simple/Chassis/Power Assisted Steering ==
  note: MOTORCYCLE
  note: VEHICLE
  note: Reverse steering direction for negative velocities
  Vx_[ms-1] : Inport
  Delta_in_[deg] : Inport  Port=2
  Constant : Constant
  Constant1 : Constant  Value=p.VehMCSwitch
  Lookup Table : Lookup  InputValues=[0 35 45 100]  Table=[1 1 0.2 0.2]
  Multiport Switch : MultiPortSwitch  Inputs=2
  Product : Product  Inputs=3  RndMeth=Zero
  Sign : Signum
  Delta_out_[deg] : Outport
  wires:
  Vx_[ms-1]/1 -> Lookup Table/1, Sign/1
  Delta_in_[deg]/1 -> Product/3
  Constant1/1 -> Multiport Switch/1
  Constant/1 -> Multiport Switch/3
  Lookup Table/1 -> Multiport Switch/2
  Multiport Switch/1 -> Product/2
  Product/1 -> Delta_out_[deg]/1
  Sign/1 -> Product/1

== system testemplanner_cs_old/Audi_A8_Sedan_2/Dynamics_Simple/Chassis/RearTyre ==
  note: alpha limiter
      | [-1 ... 1]
  note: relax_on
      | ON: 1
      | OFF: 0
  note: MOTORCYCLE ONLY
  note: VEHICLE + MOTORCYCLE
  |vx|_[ms-1] : Inport
  vy_[ms-1] : Inport  Port=2
  dpsi_[rads-1] : Inport  Port=3
  RollAngle_[rad] : Inport  Port=4
  AlphaRear : Subsystem
  Compare To Zero : simulink/Logic and Bit Operations/Compare To Zero  relop===  OutDataTypeStr=boolean  ZeroCross=off
  Configurable Subsystem : Subsystem  BlockChoice=Integrator  mask{ComputationMode=ComputationMode}
      mask prompts: ComputationMode "Computation mode:"
      mask init:
      | SetComputationMode(gcb,ComputationMode);
      settings: AttributesFormatString=%<BlockChoice>  OpenFcn=BringToFront(gcb);  MemberBlocks=Discrete-Time Integrator,Integrator
      settings: TemplateBlock=|
      | PreScanSimulinkLibrary/Configurable Subsystems/integral with reset/Configurable
      | Subsystem
  Configurable Subsystem1 : Subsystem  BlockChoice=Integrator  mask{ComputationMode=ComputationMode}
      mask prompts: ComputationMode "Computation mode:"
      mask init:
      | SetComputationMode(gcb,ComputationMode);
      settings: AttributesFormatString=%<BlockChoice>  OpenFcn=BringToFront(gcb);  MemberBlocks=Discrete-Time Integrator,Integrator
      settings: TemplateBlock=|
      | PreScanSimulinkLibrary/Configurable Subsystems/integral with reset and limits
      | for slip angle/Configurable
      | Subsystem
  Constant1 : Constant  Value=p.relax_on
  Constant2 : Constant  Value=p.relax_on
  Constant3 : Constant  Value=p.VehMCSwitch
  Data Type Conversion : DataTypeConversion  OutDataTypeStr=double
  If MC : simulink/Logic and Bit Operations/Compare To Constant  relop===  const=2  OutDataTypeStr=uint8  ZeroCross=off
  K_gamma_rear : Gain  Gain=p.Kgrear
  Linl : Fcn  Expr=(u(4) - u(5))/p.sigma_rear*u(1)
  Linl1 : Fcn  Expr=(u(4) - u(5))/p.sigma_rear*u(1)
  Mux1 : Mux  Inputs=3
  Mux2 : Mux  Inputs={3,1,1}
  Mux3 : Mux  Inputs={3,1,1}
  Prevent_instability_at_low_Vx : PreScanSimulinkLibrary/Simple_Vehicle_Dynamics/Chassis/FrontTyre/Prevent_instability_at_low_Vx  SystemSampleTime=-1  VariantActivationTime=update diagram  Latency=0  AutoFrameSizeCalculation=off
  Product : Product  RndMeth=Zero
  Sum1 : Sum  Inputs=|++
  Switch1 : Switch  Threshold=0.5  SaturateOnIntegerOverflow=on  InputSameDT=on
  Switch2 : Switch  Threshold=0.5  SaturateOnIntegerOverflow=on  InputSameDT=on
  alg.loop : Memory
  due to sign convention : Gain  Gain=-1  SaturateOnIntegerOverflow=on  OutDataTypeStr=Inherit: Same as input  ParamDataTypeStr=Inherit: Same as input
  rear_tyre : Gain  Gain=p.Krear
  FyRear_[N] : Outport
  wires:
  Prevent_instability_at_low_Vx/1 -> Switch1/3, Mux2/2
  AlphaRear/1(Alpha) -> Prevent_instability_at_low_Vx/1  "AlphaStatRear_[rad]"
  Switch1/1 -> rear_tyre/1  "AlphaRear_[rad]"
  Constant1/1 -> Switch1/2
  Sum1/1 -> FyRear_[N]/1  "FyRear_[N]"
  Mux2/1 -> Linl/1
  Linl/1 -> Configurable Subsystem1/1(In1)
  Configurable Subsystem1/1(Out1) -> Mux2/3, Switch1/1  "AlphaRelaxRear_[rad]"
  Mux1/1 -> Prevent_instability_at_low_Vx/2, AlphaRear/1(In), Mux2/1, Mux3/1
  |vx|_[ms-1]/1 -> Mux1/1, Compare To Zero/1
  vy_[ms-1]/1 -> Mux1/2
  dpsi_[rads-1]/1 -> Mux1/3
  alg.loop/1 -> Switch2/3
  Configurable Subsystem/1(Out1) -> Mux3/3, Switch2/1  "GammaRelaxRear_[rad]"
  Linl1/1 -> Configurable Subsystem/1(In1)
  Mux3/1 -> Linl1/1
  Constant2/1 -> Switch2/2
  due to sign convention/1 -> alg.loop/1, Mux3/2  "GammaStatRear_[rad]"
  RollAngle_[rad]/1 -> due to sign convention/1
  Constant3/1 -> If MC/1
  If MC/1 -> Data Type Conversion/1
  Product/1 -> Sum1/2
  Data Type Conversion/1 -> Product/2
  K_gamma_rear/1 -> Product/1
  rear_tyre/1 -> Sum1/1
  Compare To Zero/1 -> [reset]
  [reset] -> Configurable Subsystem1/2(In2)
  [reset] -> Configurable Subsystem/2(In2)
  Switch2/1 -> K_gamma_rear/1  "GammaFront_[rad]"

== system testemplanner_cs_old/Audi_A8_Sedan_2/Dynamics_Simple/Engine/Configurable Subsystem ==
  In1 : Inport
  Rate Limiter : TransferFcn  Denominator=[0.1 1]
  Out1 : Outport
  wires:
  In1/1 -> Rate Limiter/1
  Rate Limiter/1 -> Out1/1

== system testemplanner_cs_old/Audi_A8_Sedan_2/Dynamics_Simple/Engine/Configurable Subsystem1 ==
  In1 : Inport
  Integrator : Integrator  InitialCondition=p.rot_ini  LimitOutput=on  UpperSaturationLimit=p.rot_upp  LowerSaturationLimit=p.rot_low
  Out1 : Outport
  wires:
  In1/1 -> Integrator/1
  Integrator/1 -> Out1/1

== system testemplanner_cs_old/Audi_A8_Sedan_2/Dynamics_Simple/Gear: Auto Manual/If Action Subsystem ==
  In1 : Inport
  Action Port : ActionPort  PropagateVarSize=During execution  ActionPortLabel=if(u1 == 0)
  Out1 : Outport
  wires:
  In1/1 -> Out1/1

== system testemplanner_cs_old/Audi_A8_Sedan_2/Dynamics_Simple/Gear: Auto Manual/If Action Subsystem1 ==
  In1 : Inport
  Action Port : ActionPort  PropagateVarSize=During execution  ActionPortLabel=else
  Out1 : Outport
  wires:
  In1/1 -> Out1/1

== system testemplanner_cs_old/Audi_A8_Sedan_2/Dynamics_Simple/ShiftLogic/Detect Increase ==
  GearNr_[-] : Inport
  In2 : Inport  Port=2
  Constant : Constant
  Data Type Conversion : DataTypeConversion  OutDataTypeStr=double
  Data Type Conversion1 : DataTypeConversion  OutDataTypeStr=double
  Detect Increase : simulink/Logic and Bit Operations/Detect Increase  vinit=1  OutDataTypeStr=uint8
  If : If  NumInputs=2  IfExpression="u1==1 &  u2==1"
  If V0 higher of the from 2->3 shifting velocity : Subsystem  TreatAsAtomicUnit=on
  Merge : Merge
  Other : Subsystem  TreatAsAtomicUnit=on
  Out1 : Outport
  wires:
  If/2 -> Other/Action
  If V0 higher of the from 2->3 shifting velocity/1(Out1) -> Merge/1
  Other/1(Out1) -> Merge/2
  Detect Increase/1 -> Data Type Conversion/1
  Merge/1 -> Out1/1
  If/1 -> If V0 higher of the from 2->3 shifting velocity/Action
  Data Type Conversion1/1 -> If/2
  Data Type Conversion/1 -> If/1
  Constant/1 -> If V0 higher of the from 2->3 shifting velocity/1(In1)
  GearNr_[-]/1 -> Detect Increase/1
  In2/1 -> Data Type Conversion1/1, Other/1(In1)

== system testemplanner_cs_old/Audi_A8_Sedan_2/Dynamics_Simple/ShiftLogic/If Action Neutral ==
  In1 : Inport
  Action Port : ActionPort  InitializeStates=reset  PropagateVarSize=During execution  ActionPortLabel=if(u1 == 0)
  Out1 : Outport
  wires:
  In1/1 -> Out1/1

== system testemplanner_cs_old/Audi_A8_Sedan_2/Dynamics_Simple/ShiftLogic/If Action Normal ==
  In1 : Inport
  Action Port : ActionPort  InitializeStates=reset  PropagateVarSize=During execution  ActionPortLabel=else
  Out1 : Outport
  wires:
  In1/1 -> Out1/1

== system testemplanner_cs_old/Audi_A8_Sedan_2/Dynamics_Simple/ShiftLogic/If Action Reverse ==
  In1 : Inport
  Action Port : ActionPort  InitializeStates=reset  PropagateVarSize=During execution  ActionPortLabel=elseif(u1 < 0)
  Out1 : Outport
  wires:
  In1/1 -> Out1/1

== system testemplanner_cs_old/Audi_A8_Sedan_2/Dynamics_Simple/Transmission/Torque_Converter ==
  note: <= 0
  note: > 0
  note: To compensate for no hydraulic connection when in neutral gear
  nEngine_[rpm] : Inport
  nTransmission_[rpm] : Inport  Port=2
  Gear nr : Inport  Port=3
  Compare To Constant : simulink/Logic and Bit Operations/Compare To Constant  relop=<=  const=1  OutDataTypeStr=uint8  ZeroCross=off
  Compare To Zero : simulink/Logic and Bit Operations/Compare To Zero  relop=~=  OutDataTypeStr=uint8  ZeroCross=off
  Constant : Constant  Value=1/50
  Constant1 : Constant
  Constant2 : Constant
  Drag : Gain  Gain=-1
  FactorK : Lookup  InputValues=p.speedratio  Table=p.Kfactor*p.Kcorr  SaturateOnIntegerOverflow=on
  Impeller : Fcn  Expr=u^2
  Product : Product  RndMeth=Zero
  Product1 : Product  RndMeth=Zero
  Quotient : Product  Inputs=*/  InputSameDT=on  SaturateOnIntegerOverflow=on  OutDataTypeStr=Inherit: Same as first input
  SpeedRatio : Product  Inputs=*/  InputSameDT=on  SaturateOnIntegerOverflow=on  OutDataTypeStr=Inherit: Same as first input
  Sum : Sum  Inputs=|+-
  Switch : Switch  Criteria=u2 ~= 0  Threshold=0.5
  Switch1 : Switch  Criteria=u2 ~= 0
  TorqueRatio : Lookup  InputValues=[p.speedratio 1]  Table=[p.Torqueratio 0]  SaturateOnIntegerOverflow=on
  Turbine : Product  InputSameDT=on  SaturateOnIntegerOverflow=on  OutDataTypeStr=Inherit: Same as first input
  rpm2rads-1 : Gain  Gain=2*pi/60
  ImpellerTorque_[Nm] : Outport  InitialOutput=0
  TurbineTorque_[Nm] : Outport  Port=2  InitialOutput=0
  wires:
  rpm2rads-1/1 -> Quotient/1
  Turbine/1 -> Switch1/1
  TorqueRatio/1 -> Turbine/2
  Compare To Constant/1 -> Switch1/2
  Constant2/1 -> Sum/2
  Sum/1 -> Drag/1
  Drag/1 -> Switch1/3
  Product1/1 -> TurbineTorque_[Nm]/1
  Switch1/1 -> Product1/2
  Compare To Zero/1 -> Switch/2
  Gear nr/1 -> Compare To Zero/1
  Constant1/1 -> Switch/1
  Constant/1 -> Switch/3
  Switch/1 -> Product1/1, Product/1
  Product/1 -> ImpellerTorque_[Nm]/1
  Quotient/1 -> Impeller/1
  FactorK/1 -> Quotient/2
  SpeedRatio/1 -> FactorK/1, Sum/1, Compare To Constant/1, TorqueRatio/1
  Impeller/1 -> Turbine/1, Product/2
  nEngine_[rpm]/1 -> SpeedRatio/2, rpm2rads-1/1
  nTransmission_[rpm]/1 -> SpeedRatio/1
